simulink model "Copy_of_ModeloManual"  (R2022a)
settings: Solver=VariableStepAuto  StartTime=0.0  StopTime=20  RelTol=1e-3
values from neighbouring files (symbols this model uses):
  a = 0.2    [Data.m]
  b = 0.15    [Data.m]
  M = [0,0; 1,1; 6,2; 3,3; 4,4 ; 5,5]    [Data.m]
  m3 = pinv(m2)    [Data.m]
  N = 4365    [GraficasVelocidades.m]    (also in Prueba_Liapunov.m = length(p_X); WaypointsToTrayectory.m = length(X))
  R = 0.16/2    (= 0.08)    [Data.m]
  X = M(:,1)    [WaypointsToTrayectory.m]
  Y = M(:, 2)    [WaypointsToTrayectory.m]
undefined symbols (not defined in the file or in its folder): c, Z
libraries: sm_lib x35, nesl_utility x26, fl_lib x9, ee_lib x1, robotalgslib x1
(part 2 of 2)

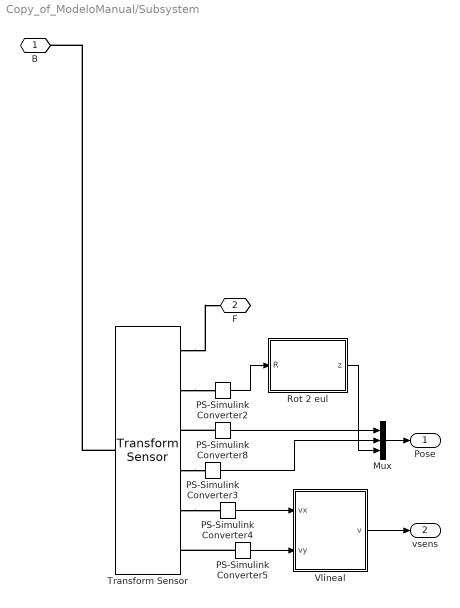
== system Copy_of_ModeloManual/Subsystem ==
  Mux : Mux  Inputs=3
  PS-Simulink Converter{2..5,8} (5 alike) : nesl_utility/PS-Simulink Converter  PhysicalDomain=network_engine_domain  SubClassName=ps_output  LeftPortType=input  RightPortType=output  PseudoPeriodic=off  Frequencies=[]  VectorFormat=inherit  Unit=inherit  AffineConversion=off
      settings: SourceProductBaseCode=SS,PW,VE
  Rot 2 eul : MATLAB Function  TreatAsAtomicUnit=on
  Transform Sensor : sm_lib/Frames and Transforms/Transform Sensor  MeasurementFrame=Base  SenseAngle=off  SenseAxis=off  SenseAngle1=off  SenseAngle2=off  SenseAngle3=off  SenseQ=off  SenseR=on  SenseOmegaX=off  SenseOmegaY=off  SenseOmegaZ=off  SenseOmega1=off  SenseOmega2=off  SenseOmega3=off  SenseQDot=off  SenseRDot=off  SenseAlphaX=off  SenseAlphaY=off  SenseAlphaZ=off  SenseAlpha1=off  SenseAlpha2=off  SenseAlpha3=off  SenseQDDot=off  SenseRDDot=off  SenseX=on  SenseY=on  SenseZ=off  SenseRad=off  SenseAzim=off  SenseDist=off  SenseInc=off  SenseXDot=on  SenseYDot=on  SenseZDot=off  SenseRadDot=off  SenseAzimDot=off  SenseDistDot=off  SenseIncDot=off  SenseXDDot=off  SenseYDDot=off  SenseZDDot=off  SenseRadDDot=off  SenseAzimDDot=off  SenseDistDDot=off  SenseIncDDot=off
  Vlineal : MATLAB Function  TreatAsAtomicUnit=on
  B : PMIOPort  Side=Left
  F : PMIOPort  Port=2  Side=Right
  Pose : Outport
  vsens : Outport  Port=2
  wires:
  Rot 2 eul/1(z) -> Mux/3
  PS-Simulink Converter2/1 -> Rot 2 eul/1(R)
  Mux/1 -> Pose/1
  Vlineal/1(v) -> vsens/1
  PS-Simulink Converter8/1 -> Mux/1
  PS-Simulink Converter3/1 -> Mux/2
  PS-Simulink Converter4/1 -> Vlineal/1(vx)
  PS-Simulink Converter5/1 -> Vlineal/2(vy)
  connections:
  Transform Sensor/RConn5 -- PS-Simulink Converter4/LConn1
  PS-Simulink Converter5/LConn1 -- Transform Sensor/RConn6
  Transform Sensor/RConn4 -- PS-Simulink Converter3/LConn1
  Transform Sensor/RConn2 -- PS-Simulink Converter2/LConn1
  PS-Simulink Converter8/LConn1 -- Transform Sensor/RConn3
  Transform Sensor/LConn1 -- B/RConn1
  Transform Sensor/RConn1 -- F/RConn1

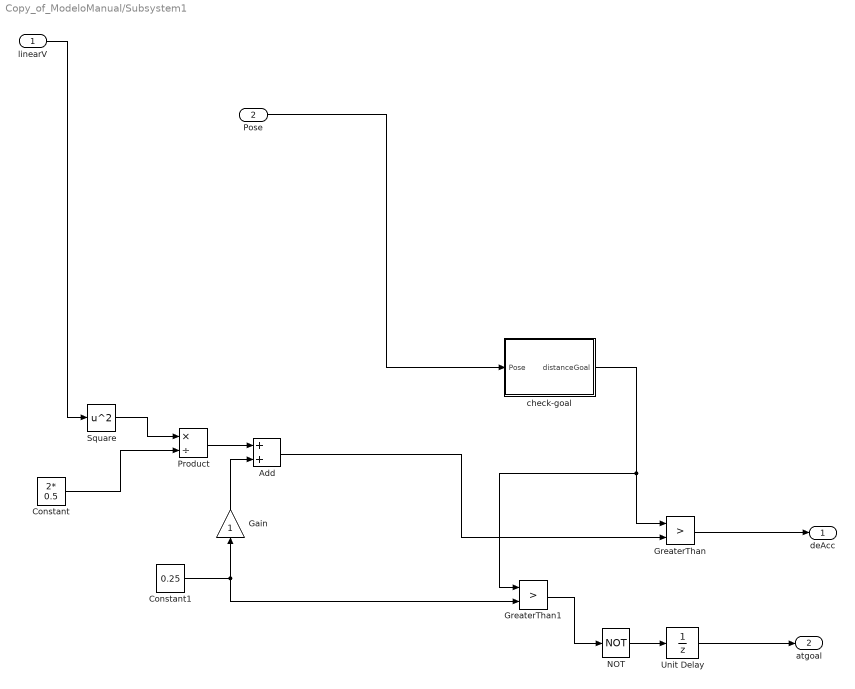
== system Copy_of_ModeloManual/Subsystem1 ==
  linearV : Inport
  Pose : Inport  Port=2
  Add : Sum
  Constant : Constant  Value=2* 0.5
  Constant1 : Constant  Value=0.25
  Gain : Gain
  GreaterThan : RelationalOperator  Operator=>  OutDataTypeStr=boolean  RndMeth=Simplest  InputSameDT=off
  GreaterThan1 : RelationalOperator  Operator=>  OutDataTypeStr=boolean  RndMeth=Simplest  InputSameDT=off
  NOT : Logic  Operator=NOT  IconShape=distinctive  AllPortsSameDT=off  OutDataTypeStr=boolean
  Product : Product  Inputs=*/
  Square : Math  Operator=square
  Unit Delay : UnitDelay  SampleTime=-1  HasFrameUpgradeWarning=on
  check-goal : Subsystem
  deAcc : Outport
  atgoal : Outport  Port=2
  wires:
  check-goal/1(distanceGoal) -> GreaterThan1/1, GreaterThan/1
  Constant/1 -> Product/2
  Constant1/1 -> GreaterThan1/2, Gain/1
  Add/1 -> GreaterThan/2
  Product/1 -> Add/1
  GreaterThan1/1 -> NOT/1
  Square/1 -> Product/1
  GreaterThan/1 -> deAcc/1
  NOT/1 -> Unit Delay/1
  Pose/1 -> check-goal/1(Pose)
  Unit Delay/1 -> atgoal/1
  linearV/1 -> Square/1
  Gain/1 -> Add/2

== system Copy_of_ModeloManual/Tapa ==
  DegTa : fl_lib/Physical Signals/Sources/PS Constant  constant=0 rad/s
      settings: SourceProductBaseCode=PW,SS,VE
  Int-Tapa : sm_lib/Frames and Transforms/Rigid Transform  TranslationMethod=Cartesian  TranslationStandardOffset=0  TranslationLengthUnit=mm  TranslationStandardAxis=+Z  TranslationCartesianOffset=[177 140 12.5]  TranslationROffset=0  TranslationROffsetUnits=m  TranslationZOffset=0  TranslationZOffsetUnits=m  TranslationThetaOffset=0  TranslationThetaOffsetUnits=deg  RotationMethod=StandardAxis  RotationAngleUnits=deg  RotationStandardAxis=+X  RotationAngle=90  RotationArbitraryAxis=[0 0 1]  FollAlignAxisA=+X  BaseAlignAxisA=+Y  FollAlignAxisB=+Y  BaseAlignAxisB=+Z  RotationSequenceAxes=FollowerAxes  RotationSequence=XYX  RotationSequenceAngles=[0 0 0]  RotationSequenceAnglesUnits=deg  RotationMatrix=[1 0 0; 0 1 0; 0 0 1]
  PS Integrator : fl_lib/Physical Signals/Linear Operators/PS Integrator  reset_method=foundation.enum.IntegratorResetSpec.None  initial_condition_spec=foundation.enum.IntegratorICSpec.Internal  x0=0 rad
      settings: SourceProductBaseCode=PW,SS,VE
  PS Saturation : fl_lib/Physical Signals/Nonlinear Operators/PS Saturation  upper_limit=0 rad  lower_limit=-pi/2 rad
      settings: SourceProductBaseCode=PW,SS,VE
  Servo-Tapa : sm_lib/Joints/Revolute Joint  JointMode=Normal  SenseConstraintForce=off  SenseConstraintForceX=off  SenseConstraintForceY=off  SenseConstraintForceZ=off  SenseConstraintTorque=off  SenseConstraintTorqueX=off  SenseConstraintTorqueY=off  SenseConstraintTorqueZ=off  SenseTotalForce=off  SenseTotalForceX=off  SenseTotalForceY=off  SenseTotalForceZ=off  SenseTotalTorque=off  SenseTotalTorqueX=off  SenseTotalTorqueY=off  SenseTotalTorqueZ=off  CompositeWrenchDir=FollowerOnBase  CompositeWrenchFrame=BaseFrame  EquilibriumPosition=0  EquilibriumPositionUnits=deg  SpringStiffness=0  SpringStiffnessUnits=N*m/deg  DampingCoefficient=0  DampingCoefficientUnits=N*m/(deg/s)  TorqueActuationMode=ComputedTorque  MotionActuationMode=InputMotion  SensePosition=off  SenseVelocity=off  SenseAcceleration=off  SenseTorqueForce=off  SenseLowerLimitTorqueForce=off  SenseUpperLimitTorqueForce=off  LowerLimitSpecify=on  LowerLimitBound=-pi/2  LowerLimitBoundUnits=deg  LowerLimitStiffness=1e4  LowerLimitStiffnessUnits=N*m/deg  LowerLimitDamping=10  LowerLimitDampingUnits=N*m/(deg/s)  LowerLimitTransitionRegionWidth=0.1  LowerLimitTransitionRegionWidthUnits=deg  UpperLimitSpecify=on  UpperLimitBound=0  UpperLimitBoundUnits=deg  UpperLimitStiffness=1e4  UpperLimitStiffnessUnits=N*m/deg  UpperLimitDamping=10  UpperLimitDampingUnits=N*m/(deg/s)  UpperLimitTransitionRegionWidth=0.1  UpperLimitTransitionRegionWidthUnits=deg  PositionTargetSpecify=off  PositionTargetPriority=High  PositionTargetValue=0  PositionTargetValueUnits=deg  VelocityTargetSpecify=off  VelocityTargetPriority=High  VelocityTargetValue=0  VelocityTargetValueUnits=deg/s
  TAPA Solid : sm_lib/Body Elements/File Solid  ExtGeomFileName=TapaOriented_ipt_dee1459.STEP  UnitType=FromFile  ExtGeomFileUnits=m  StepReaderType=HEX  ExportConvexHullGeometry=off  InertiaType=CalculateFromGeometry  Mass=2  MassUnits=kg  CenterOfMass=[0 0 0]  CenterOfMassUnits=m  MomentsOfInertia=[1 1 1]  MomentsOfInertiaUnits=kg*m^2  ProductsOfInertia=[0 0 0]  ProductsOfInertiaUnits=kg*m^2  BasedOnType=Mass  Density=1000  DensityUnits=kg/m^3  DoExposeReferenceFrame=on  SerializedFrames=<Frames/>  GraphicType=FromGeometry  MarkerShape=Sphere  MarkerSize=10  GraphicVisPropType=SimpleVisualProperties  GraphicDiffuseColor=[0.5 0.5 0.5]  GraphicSpecularColor=[0.5 0.5 0.5 1.0]  GraphicAmbientColor=[0.15 0.15 0.15 1.0]  GraphicEmissiveColor=[0.0 0.0 0.0 1.0]  GraphicShininess=75  GraphicOpacity=1.0
  Ch : PMIOPort  Side=Left
  connections:
  TAPA Solid/RConn1 -- Int-Tapa/LConn1
  Int-Tapa/RConn1 -- Servo-Tapa/RConn1
  Servo-Tapa/LConn1 -- Ch/RConn1
  PS Integrator/LConn1 -- DegTa/RConn1
  PS Saturation/RConn1 -- Servo-Tapa/LConn2
  PS Saturation/LConn1 -- PS Integrator/RConn1

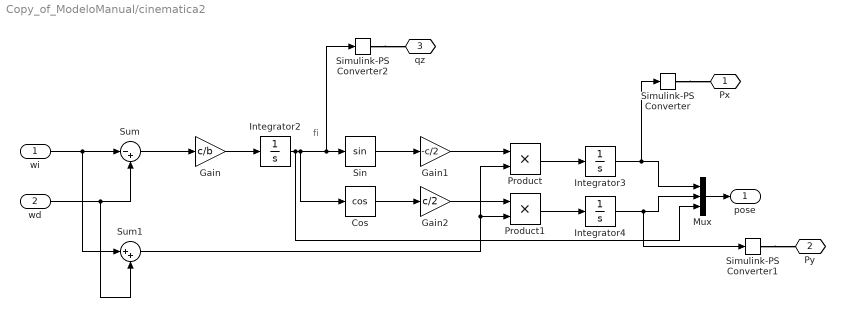
== system Copy_of_ModeloManual/cinematica2 ==
  note: fi
  wi : Inport
  wd : Inport  Port=2
  Cos : Trigonometry  Operator=cos
  Gain : Gain  Gain=c/b
  Gain1 : Gain  Gain=-c/2
  Gain2 : Gain  Gain=c/2
  Integrator2 : Integrator
  Integrator3 : Integrator
  Integrator4 : Integrator
  Mux : Mux  Inputs=3
  Product : Product
  Product1 : Product
  Simulink-PS Converter : nesl_utility/Simulink-PS Converter  PhysicalDomain=network_engine_domain  SubClassName=ps_input  LeftPortType=input  RightPortType=output  PseudoPeriodic=off  Frequencies=[]  NoiseDistribution=none  NoiseParameters=[]  Unit=m  AffineConversion=off  FilteringAndDerivatives=filter  SimscapeFilterOrder=2  InputFilterTimeConstant=0.001  UdotUserProvided=0
      settings: SourceProductBaseCode=SS,PW,VE
  Simulink-PS Converter1 : nesl_utility/Simulink-PS Converter  PhysicalDomain=network_engine_domain  SubClassName=ps_input  LeftPortType=input  RightPortType=output  PseudoPeriodic=off  Frequencies=[]  NoiseDistribution=none  NoiseParameters=[]  Unit=m  AffineConversion=off  FilteringAndDerivatives=filter  SimscapeFilterOrder=2  InputFilterTimeConstant=0.001  UdotUserProvided=0
      settings: SourceProductBaseCode=SS,PW,VE
  Simulink-PS Converter2 : nesl_utility/Simulink-PS Converter  PhysicalDomain=network_engine_domain  SubClassName=ps_input  LeftPortType=input  RightPortType=output  PseudoPeriodic=off  Frequencies=[]  NoiseDistribution=none  NoiseParameters=[]  Unit=rad  AffineConversion=off  FilteringAndDerivatives=filter  SimscapeFilterOrder=2  InputFilterTimeConstant=0.001  UdotUserProvided=0
      settings: SourceProductBaseCode=SS,PW,VE
  Sin : Trigonometry
  Sum : Sum  Inputs=|-+
  Sum1 : Sum  Inputs=|++
  Px : PMIOPort  Side=Right
  Py : PMIOPort  Port=2  Side=Right
  qz : PMIOPort  Port=3  Side=Right
  pose : Outport
  wires:
  Sum1/1 -> Product1/2, Product/2
  Gain1/1 -> Product/1
  wi/1 -> Sum1/1, Sum/1
  wd/1 -> Sum1/2, Sum/2
  Product/1 -> Integrator3/1
  Cos/1 -> Gain2/1
  Gain/1 -> Integrator2/1
  Sum/1 -> Gain/1
  Product1/1 -> Integrator4/1
  Sin/1 -> Gain1/1
  Gain2/1 -> Product1/1
  Integrator3/1 -> Simulink-PS Converter/1, Mux/1
  Mux/1 -> pose/1
  Integrator4/1 -> Simulink-PS Converter1/1, Mux/2
  Integrator2/1 -> Mux/3, Cos/1, Simulink-PS Converter2/1, Sin/1
  connections:
  Simulink-PS Converter/RConn1 -- Px/RConn1
  Simulink-PS Converter1/RConn1 -- Py/RConn1
  Simulink-PS Converter2/RConn1 -- qz/RConn1

== system Copy_of_ModeloManual/hold ==
  deAcc : Inport
  Constant9 : Constant  Value=inf
  NOT1 : Logic  Operator=NOT  IconShape=distinctive  AllPortsSameDT=off  OutDataTypeStr=boolean
  RoverStopTime : Subsystem
  Switch3 : Switch  Criteria=u2 > Threshold  SaturateOnIntegerOverflow=off  InputSameDT=off
  Unit Delay1 : UnitDelay  SampleTime=-1  HasFrameUpgradeWarning=on
  deaccelStartTime : Outport
  wires:
  Unit Delay1/1 -> Switch3/2
  RoverStopTime/1(DeAccelTime) -> Switch3/1
  Switch3/1 -> deaccelStartTime/1
  NOT1/1 -> RoverStopTime/1(Enable), Unit Delay1/1
  Constant9/1 -> Switch3/3
  deAcc/1 -> NOT1/1

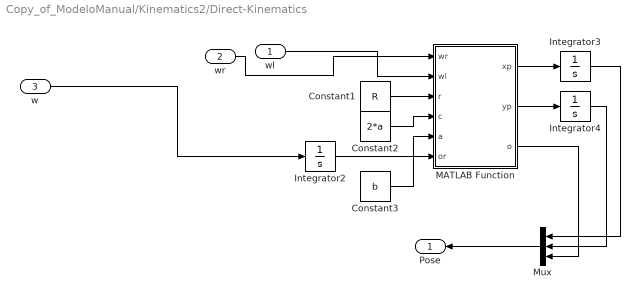
== system Copy_of_ModeloManual/Kinematics2/Direct-Kinematics ==
  wl : Inport
  wr : Inport  Port=2
  w : Inport  Port=3
  Constant1 : Constant  Value=R
  Constant2 : Constant  Value=2*a
  Constant3 : Constant  Value=b
  Integrator2 : Integrator
  Integrator3 : Integrator
  Integrator4 : Integrator
  MATLAB Function : MATLAB Function  TreatAsAtomicUnit=on
  Mux : Mux  Inputs=3
  Pose : Outport
  wires:
  Integrator4/1 -> Mux/2
  Constant3/1 -> MATLAB Function/5(a)
  MATLAB Function/3(o) -> Mux/3
  MATLAB Function/1(xp) -> Integrator3/1
  Integrator3/1 -> Mux/1
  Integrator2/1 -> MATLAB Function/6(or)
  w/1 -> Integrator2/1
  wr/1 -> MATLAB Function/1(wr)
  Constant1/1 -> MATLAB Function/3(r)
  MATLAB Function/2(yp) -> Integrator4/1
  Constant2/1 -> MATLAB Function/4(c)
  Mux/1 -> Pose/1
  wl/1 -> MATLAB Function/2(wl)

== system Copy_of_ModeloManual/Kinematics2/Inverse-Kinematics ==
  v : Inport
  w : Inport  Port=2
  Gain : Gain  Gain=b/2
  Gain1 : Gain  Gain=1/R
  Gain2 : Gain  Gain=1/R
  Sum : Sum  Inputs=|+-
  Sum1 : Sum  Inputs=|++
  wL : Outport
  wR : Outport  Port=2
  wires:
  Gain/1 -> Sum1/2, Sum/2
  Sum/1 -> Gain1/1
  Gain1/1 -> wL/1
  Gain2/1 -> wR/1
  v/1 -> Sum1/1, Sum/1
  Sum1/1 -> Gain2/1
  w/1 -> Gain/1

== system Copy_of_ModeloManual/Subsystem1/check-goal ==
  Pose : Inport
  Constant : Constant  Value=[5,5]
  MATLAB Function : MATLAB Function  TreatAsAtomicUnit=on
  Scope : Scope
  Selector : Selector  InputPortWidth=3  IndexOptions=Index vector (dialog)  Indices=[1 2]  OutputSizes=1
  distanceGoal : Outport
  wires:
  Pose/1 -> Selector/1
  Selector/1 -> MATLAB Function/1(posexy)
  Constant/1 -> MATLAB Function/2(goal)
  MATLAB Function/1(distanceGoal) -> distanceGoal/1, Scope/1

== system Copy_of_ModeloManual/hold/RoverStopTime ==
  Enable : Inport
  Clock : Clock
  Constant2 : Constant
  Display : Display
  Enabled Subsystem1 : Subsystem  TreatAsAtomicUnit=on
      settings: MinAlgLoopOccurrences=on
  Switch : Switch  Criteria=u2 > Threshold  SaturateOnIntegerOverflow=off  InputSameDT=off
  Unit Delay : UnitDelay  SampleTime=-1  HasFrameUpgradeWarning=on
  DeAccelTime : Outport
  wires:
  Enabled Subsystem1/1(Out1) -> Switch/2
  Enable/1 -> Enabled Subsystem1/Enable
  Switch/1 -> Unit Delay/1
  Unit Delay/1 -> Display/1, DeAccelTime/1, Switch/1
  Clock/1 -> Switch/3
  Constant2/1 -> Enabled Subsystem1/1(In1)

== system Copy_of_ModeloManual/hold/RoverStopTime/Enabled Subsystem1 ==
  In1 : Inport
  Enable : EnablePort
  Out1 : Outport
  wires:
  In1/1 -> Out1/1

== matlab function Copy_of_ModeloManual/Subsystem1/check-goal/MATLAB Function ==
  data: posexy input; distanceGoal output; goal input
function distanceGoal  = fcn( posexy, goal)

distanceGoal = sqrt(((goal(1)-posexy(1))^2)+ ((goal(2)-posexy(2))^2) );
end

== matlab function Copy_of_ModeloManual/Subsystem/Rot 2 eul ==
  data: z output; R input
function z  = fcn(R)
out = rotm2eul(R);
z = out(1);
end

== matlab function Copy_of_ModeloManual/Subsystem/Vlineal ==
  data: vx input; v output; vy input
function v = fcn(vx, vy)

v = sqrt((vx)^2 + (vy)^2);
end

== matlab function Copy_of_ModeloManual/Kinematics2/Direct-Kinematics/MATLAB Function ==
  data: xp output; yp output; wr input; wl input; r input; c input; a input; o output; or input
function [xp,yp,o] = fcn(wr,wl,r,c,a,or)

o= or;

v1= c*cos(o) - 2*a*sin(o);
v2= c*cos(o) + 2*a*sin(o);
v3= c*sin(o) + 2*a*cos(o);
v4= c*sin(o) - 2*a*cos(o);

xp=(r/(2*c))*(v1*wr+v2*wl);
yp=(r/(2*c))*(v3*wr+v4*wl);

== matlab function Copy_of_ModeloManual/Trapezoidal Vel Profile ==
  data: linVel input; t input; t1 input; lin_Vel_out output; accel input; deaccelStartTime input
function lin_Vel_out = fcn(linVel,t,t1,accel,deaccelStartTime)
% Function to create a trapezoidal profile for rover's desired linear
% velocity

t2 = linVel/accel + t1;
t3 = deaccelStartTime + 0.2;
tf = linVel/accel + t3;

if t>=t1 && t<t2 
    lin_Vel_out = accel*(t-t1);

elseif t>=t2 && t < t3 
    lin_Vel_out = linVel;

elseif t>= t3 && t < tf 
    lin_Vel_out = linVel-accel*(t-t3);

else
    lin_Vel_out = 0;    
end


end
